simulink library "fixptlib"  (Simulink 4.00)
libraries: fixpt_lib_3p1 x25
settings Model: RequirementInfo=9  Creator=andyb  LastModifiedBy=andyb  ExtModeAutoUpdateStatusClock=off

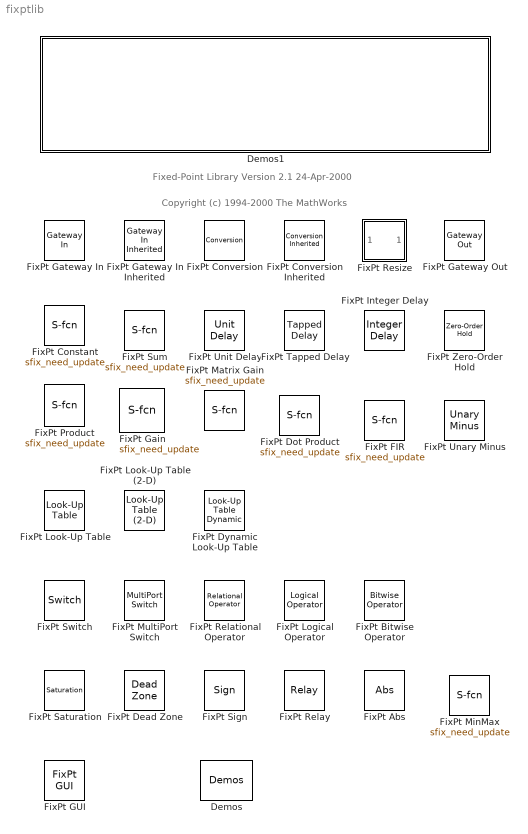
== system fixptlib ==
  note: Fixed-Point Library Version 2.1
      | 24-Apr-2000
  note: Copyright (c) 1994-2000 The MathWorks
  Demos : fixpt_lib_3p1/Demos
  Demos1 : Subsystem
      settings: OpenFcn=fixpt;  RTWFcnNameOpts=Auto  RTWFileNameOpts=Auto
      mask Display: disp('Obsolete version of Fixed-Point Blockset library.\n\nDouble Click this block to execute FIXPT.\n\nFIXPT will open latest version of the library.')
  FixPt Abs : fixpt_lib_3p1/Math/Abs  DoSatur=off
  FixPt Bitwise Operator : fixpt_lib_3p1/Bits/Bitwise Operator  logicop=AND  UseBitMask=on  BitMask=2^5+2^2+2^0  BitMaskRealWorld=Stored Integer
  FixPt Constant : S-Function  FunctionName=sfix_need_update  Parameters=NumInputs  PortCounts=[]  SFunctionModules=''  mask(Fixed-Point Constant (Obsolete)){constval=0.0, OutDataType=sfix(16), OutScaling=2^-1000, ConRadixGroup=Best Precision: Vector-wise, DblOver=off, SpecifyOutputDataType=on, SpecifyOutputScaling=on}
      mask prompts: constval "Constant value:"; OutDataType "Output data type:     ex.  sfix(16),  uint(8),  float('single')"; OutScaling "Output scaling:    Slope or [Slope Bias]    ex.  2^-9"; ConRadixGroup "Output scaling:"; DblOver "Override data type(s) with doubles"; SpecifyOutputDataType "Specify Output Data Type (otherwise inherit) ..."; SpecifyOutputScaling "Specify Output Scaling (otherwise inherit) ..."
      mask help:
      | Generate a constant value.
      |
      | This block is obsolete and is not compatible with the current version of Fixed Point Blockset.  The block needs to be replaced using FIXPT_UPDATE.
      mask init:
      | NumInputs = ~SpecifyOutputDataType | ~SpecifyOutputScaling;
      mask Help: This block is obsolete and is not compatible with the current version of Fixed Point Blockset.  The block needs to be replaced using FIXPT_UPDATE.
      mask StyleString: edit,edit,edit,popup(Use Specified Scaling|Best Precision: Vector-wise),checkbox,checkbox,checkbox
      mask CallbackString: fixptdialog(gcbh)|fixptdialog(gcbh)||fixptdialog(gcbh)|||
      mask Display:
      | disp(fixpt_mask_disp_prep(constval))
      | patch([2 2 10 10 4 4 8 8 4 4 2 ],[2 10 10 8 8 6 6 4 4 2 2 ],[0 0 0],'bottom-right');
  FixPt Conversion : fixpt_lib_3p1/Data Type/Conversion  ConvertRealWorld=Real World Value  OutputDataTypeScalingMode=Specify via dialog  OutDataType=sfix(16)  OutScaling=2^-10  DoSatur=off  DblOver=off  dolog=on
  FixPt Conversion Inherited : fixpt_lib_3p1/Data Type/Conversion Inherited  ConvertRealWorld=Real World Value  DoSatur=off  DblOver=off  dolog=on
  FixPt Dead Zone : fixpt_lib_3p1/Nonlinear/Dead Zone  UpperValue=1  LowerValue=-1  DoSatur=off
  FixPt Dot Product : S-Function  FunctionName=sfix_need_update  Parameters=2  PortCounts=[]  SFunctionModules=''  mask(Fixed-Point Dot Product (Obsolete)){OutDataType=sfix(16), OutScaling=2^-10, LockScale=off, RndMeth=Floor, DoSatur=off, DblOver=off, dolog=on, SpecifyOutputDataTypeAndScaling=on}
      mask prompts: OutDataType "Output data type:     ex.  sfix(16),  uint(8),  float('single')"; OutScaling "Output scaling:    Slope or [Slope Bias]    ex.  2^-9"; LockScale "Lock output scaling so autoscaling tool can't change it"; RndMeth "Round toward:"; DoSatur "Saturate to max or min when overflows occur"; DblOver "Override data type(s) with doubles"; dolog "Log minimums and maximums"
      mask help:
      | Inner (dot) product.
      | y = sum(conj(u1).*u2)
      |
      | This block is obsolete and is not compatible with the current version of Fixed Point Blockset.  The block needs to be replaced using FIXPT_UPDATE.
      mask Help: This block is obsolete and is not compatible with the current version of Fixed Point Blockset.  The block needs to be replaced using FIXPT_UPDATE.
      mask StyleString: edit,edit,checkbox,popup(Zero|Nearest|Ceiling|Floor),checkbox,checkbox,checkbox,checkbox
      mask CallbackString: fixptdialog(gcbh)|||||||
      mask Display:
      | patch([0.55 0.5433 0.525 0.5 0.475 0.4567 0.45 0.4567 0.475 0.5 0.525 0.5433 0.55],[ 0.5 0.525 0.5433 0.55 0.5433 0.525 0.5 0.475 0.4567 0.45 0.4567 0.475 0.5],[0 0 0])
      | patch([2 2 10 10 4 4 8 8 4 4 2 ],[2 10 10 8 8 6 6 4 4 2 2 ],[0 0 0],'bottom-right');
  FixPt Dynamic Look-Up Table : fixpt_lib_3p1/LookUp/Look-Up Table Dynamic  LookUpMeth=Interpolation-Use End Values  OutputDataTypeScalingMode=Specify via dialog  OutDataType=sfix(16)  OutScaling=2^-10  DoSatur=off  DblOver=off  dolog=on
  FixPt FIR : S-Function  FunctionName=sfix_need_update  Parameters=1  PortCounts=[]  SFunctionModules=''  mask(Fixed-Point FIR (Obsolete)){mgainval=[0.1:0.1:1 0.9:-0.1:0.1], vinit=0.0, samptime=-1, GainDataType=sfix( 16 ), GainScaling=2^-14, MatRadixGroup=Best Precision: Matrix-wise, OutDataType=sfix(16), OutScaling=2^-10, LockScale=off, RndMeth=Floor, DoSatur=off, DblOver=off, dolog=on, SpecifyOutputDataTypeAndScaling=on}
      mask prompts: mgainval "FIR coefficients:"; vinit "Initial condition:"; samptime "Sample time:"; GainDataType "Parameter data type:     ex. sfix(16),  uint(8), float('single')"; GainScaling "Parameter scaling:    Slope    ex.  2^-9"; MatRadixGroup "Parameter scaling:"; OutDataType "Output data type:     ex.  sfix(16),  uint(8),  float('single')"; OutScaling "Output scaling:    Slope or [Slope Bias]    ex.  2^-9"; LockScale "Lock output scaling so autoscaling tool can't change it"; RndMeth "Round toward:"; DoSatur "Saturate to max or min when overflows occur"; DblOver "Override data type(s) with doubles"; dolog "Log minimums and maximums"
      mask help:
      | Implement a finite impulse response (FIR) filter.
      |
      | This block is obsolete and is not compatible with the current version of Fixed Point Blockset.  The block needs to be replaced using FIXPT_UPDATE.
      mask init:
      | if MatRadixGroup == 5
      |     RadixGroup = 1; % BEST_PREC_MAT
      | elseif MatRadixGroup == 4
      |     RadixGroup = 2; % BEST_PREC_COL
      | elseif MatRadixGroup == 3
      |     RadixGroup = 3; % BEST_PREC_ROW
      | elseif MatRadixGroup == 2
      |     RadixGroup = 4; % BEST_PREC_ELE
      | else
      |     RadixGroup = 0; % BEST_PREC_OFF
      | end
      mask Help: This block is obsolete and is not compatible with the current version of Fixed Point Blockset.  The block needs to be replaced using FIXPT_UPDATE.
      mask StyleString: edit,edit,edit,edit,edit,popup(Use Specified Scaling|Best Precision: Element-wise|Best Precision: Row-wise|Best Precision: Column-wise|Best Precision: Matrix-wise),edit,edit,checkbox,popup(Zero|Nearest|Ceiling|Floor),checkbox,checkbox,checkbox,checkbox
      mask CallbackString: fixptdialog(gcbh)|||fixptdialog(gcbh)||fixptdialog(gcbh)|fixptdialog(gcbh)|||||||
      mask Display:
      | fprintf(fixpt_fir_mask_data(mgainval,'dispstr'))
      | plot(fixpt_fir_mask_data(mgainval,1),fixpt_fir_mask_data(mgainval,0))
      | patch([2 2 10 10 4 4 8 8 4 4 2 ],[2 10 10 8 8 6 6 4 4 2 2 ],[0 0 0],'bottom-right');
  FixPt GUI : fixpt_lib_3p1/FixPt GUI
  FixPt Gain : S-Function  FunctionName=sfix_need_update  Parameters=1  PortCounts=[]  SFunctionModules=''  mask(Fixed-Point Gain (Obsolete)){gainval=1.0, GainDataType=sfix( 16 ), GainScaling=2^-14, VecRadixGroup=Best Precision: Matrix-wise, OutDataType=sfix(16), OutScaling=2^-10, LockScale=off, RndMeth=Floor, DoSatur=off, DblOver=off, dolog=on, ElevsMatrix=Element-wise(K.*u), SpecifyOutputDataTypeAndScaling=on}
      mask prompts: gainval "Gain value:"; GainDataType "Parameter data type:     ex. sfix(16),  uint(8), float('single')"; GainScaling "Parameter scaling:    Slope    ex.  2^-9"; VecRadixGroup "Parameter scaling:"; OutDataType "Output data type:     ex.  sfix(16),  uint(8),  float('single')"; OutScaling "Output scaling:    Slope or [Slope Bias]    ex.  2^-9"; LockScale "Lock output scaling so autoscaling tool can't change it"; RndMeth "Round toward:"; DoSatur "Saturate to max or min when overflows occur"; DblOver "Override data type(s) with doubles"; dolog "Log minimums and maximums"; ElevsMatrix "Multiplication"
      mask help:
      | Multiply the input by a constant (gain).
      |
      | This block is obsolete and is not compatible with the current version of Fixed Point Blockset.  The block needs to be replaced using FIXPT_UPDATE.
      mask init:
      | if VecRadixGroup >= 5
      |     RadixGroup = 1; % BEST_PREC_MAT
      | elseif VecRadixGroup == 4
      |     RadixGroup = 2; % BEST_PREC_COL
      | elseif VecRadixGroup == 3
      |     RadixGroup = 3; % BEST_PREC_ROW
      | elseif VecRadixGroup == 2
      |     RadixGroup = 4; % BEST_PREC_ELE
      | else
      |     RadixGroup = 0; % BEST_PREC_OFF
      | end
      mask Help: This block is obsolete and is not compatible with the current version of Fixed Point Blockset.  The block needs to be replaced using FIXPT_UPDATE.
      mask StyleString: edit,edit,edit,popup(Use Specified Scaling|Best Precision: Element-wise|Best Precision: Row-wise|Best Precision: Column-wise|Best Precision: Matrix-wise|Best Precision: Vector-wise),edit,edit,checkbox,popup(Zero|Nearest|Ceiling|Floor),checkbox,checkbox,checkbox,popup(Element-wise(K.*u)|Matrix(K*u)|Matrix(u*K)|Matrix(K*u) (u vector)),checkbox
      mask CallbackString: fixptdialog(gcbh)|fixptdialog(gcbh)||fixptdialog(gcbh)|fixptdialog(gcbh)||||||||
      mask Display:
      | disp(fixpt_mask_disp_prep(gainval))
      | plot(fixpt_gain_mask_data(gcbh,1),fixpt_gain_mask_data(gcbh,0))
      | patch([2 2 10 10 4 4 8 8 4 4 2 ],[2 10 10 8 8 6 6 4 4 2 2 ],[0 0 0],'bottom-right');
  FixPt Gateway In : fixpt_lib_3p1/Data Type/Gateway In  InRealWorld=Real World Value  OutputDataTypeScalingMode=Specify via dialog  OutDataType=sfix(16)  OutScaling=2^-10  DoSatur=off  DblOver=off  dolog=on
  FixPt Gateway In Inherited : fixpt_lib_3p1/Data Type/Gateway In Inherited  InRealWorld=Real World Value  DoSatur=off  DblOver=off  dolog=on
  FixPt Gateway Out : fixpt_lib_3p1/Data Type/Gateway Out  OutRealWorld=Real World Value  OutBuiltInType=double  DoSatur=off  dolog=off
  FixPt Integer Delay : fixpt_lib_3p1/Delays & Holds/Integer Delay  vinit=0.0  samptime=-1  NumDelays=4
  FixPt Logical Operator : fixpt_lib_3p1/Logic & Comparison/Logical Operator  logicop=AND  NumInputPorts=2  LogicDataType=uint(8)
  FixPt Look-Up Table : fixpt_lib_3p1/LookUp/Look-Up Table  XLookUpData=-5:5  YLookUpData=tanh([-5:5])  LookUpMeth=Interpolation-Use End Values  OutputDataTypeScalingMode=Specify via dialog  OutDataType=sfix(16)  OutScaling=2^-10  DoSatur=off  DblOver=off  dolog=on
  FixPt Look-Up Table (2-D) : fixpt_lib_3p1/LookUp/Look-Up Table (2-D)  RowLookUpData=[1:3]  ColLookUpData=[1:3]  TableLookUpData=[4 5 6;16 19 20;10 18 23]  LookUpMeth=Interpolation-Use End Values  OutputDataTypeScalingMode=Specify via dialog  OutDataType=sfix(16)  OutScaling=2^-10  DoSatur=off  DblOver=off  dolog=on
  FixPt Matrix Gain : S-Function  FunctionName=sfix_need_update  Parameters=1  PortCounts=[]  SFunctionModules=''  mask(Fixed-Point Matrix Gain (Obsolete)){mgainval=eye(3,3), GainDataType=sfix( 16 ), GainScaling=2^-14, MatRadixGroup=Best Precision: Matrix-wise, OutDataType=sfix(16), OutScaling=2^-10, LockScale=off, RndMeth=Floor, DoSatur=off, DblOver=off, dolog=on, ElevsMatrix=Matrix(K*u) (u vector), SpecifyOutputDataTypeAndScaling=on}
      mask prompts: mgainval "Gain matrix value:"; GainDataType "Parameter data type:     ex. sfix(16),  uint(8), float('single')"; GainScaling "Parameter scaling:    Slope    ex.  2^-9"; MatRadixGroup "Parameter scaling:"; OutDataType "Output data type:     ex.  sfix(16),  uint(8),  float('single')"; OutScaling "Output scaling:    Slope or [Slope Bias]    ex.  2^-9"; LockScale "Lock output scaling so autoscaling tool can't change it"; RndMeth "Round toward:"; DoSatur "Saturate to max or min when overflows occur"; DblOver "Override data type(s) with doubles"; dolog "Log minimums and maximums"; ElevsMatrix "Multiplication"
      mask help:
      | Multiply the input by a constant (gain).
      |
      | This block is obsolete and is not compatible with the current version of Fixed Point Blockset.  The block needs to be replaced using FIXPT_UPDATE.
      mask init: same as fixptlib/FixPt FIR
      mask Help: This block is obsolete and is not compatible with the current version of Fixed Point Blockset.  The block needs to be replaced using FIXPT_UPDATE.
      mask StyleString: edit,edit,edit,popup(Use Specified Scaling|Best Precision: Element-wise|Best Precision: Row-wise|Best Precision: Column-wise|Best Precision: Matrix-wise),edit,edit,checkbox,popup(Zero|Nearest|Ceiling|Floor),checkbox,checkbox,checkbox,popup(Element-wise(K.*u)|Matrix(K*u)|Matrix(u*K)|Matrix(K*u) (u vector)),checkbox
      mask CallbackString: fixptdialog(gcbh)|fixptdialog(gcbh)||fixptdialog(gcbh)|fixptdialog(gcbh)||||||||
      mask Display:
      | fprintf('K')
      | patch([2 2 10 10 4 4 8 8 4 4 2 ],[2 10 10 8 8 6 6 4 4 2 2 ],[0 0 0],'bottom-right');
  FixPt MinMax : S-Function  FunctionName=sfix_need_update  Parameters=Inputs  PortCounts=[]  SFunctionModules=''  mask(Fixed-Point MinMax (Obsolete)){Function=min, Inputs=1, OutDataType=sfix(16), OutScaling=2^-10, LockScale=off, RndMeth=Floor, DoSatur=off, DblOver=off, dolog=on, SpecifyOutputDataTypeAndScaling=on}
      mask prompts: Inputs "Number of input ports:"; OutDataType "Output data type:     ex.  sfix(16),  uint(8),  float('single')"; OutScaling "Output scaling:    Slope or [Slope Bias]    ex.  2^-9"; LockScale "Lock output scaling so autoscaling tool can't change it"; RndMeth "Round toward:"; DoSatur "Saturate to max or min when overflows occur"; DblOver "Override data type(s) with doubles"; dolog "Log minimums and maximums"
      mask help:
      | Output min or max of input.  For a single input, operators are applied across the input vector.  For multiple inputs, operators are applied across the inputs.
      |
      | This block is obsolete and is not compatible with the current version of Fixed Point Blockset.  The block needs to be replaced using FIXPT_UPDATE.
      mask Help: This block is obsolete and is not compatible with the current version of Fixed Point Blockset.  The block needs to be replaced using FIXPT_UPDATE.
      mask StyleString: popup(min|max),edit,edit,edit,checkbox,popup(Zero|Nearest|Ceiling|Floor),checkbox,checkbox,checkbox,checkbox
      mask CallbackString: ||fixptdialog(gcbh)|||||||
      mask Display:
      | disp(char((Function==1)*'min'+(Function==2)*'max'))
      | patch([2 2 10 10 4 4 8 8 4 4 2 ],[2 10 10 8 8 6 6 4 4 2 2 ],[0 0 0],'bottom-right');
  FixPt MultiPort Switch : fixpt_lib_3p1/Select/MultiPort Switch  NumInputPorts=3  zeroidx=off  DoSatur=off  dolog=on
  FixPt Product : S-Function  FunctionName=sfix_need_update  Parameters=length(mulstr)  PortCounts=[]  SFunctionModules=''  mask(Fixed-Point Product (Obsolete)){listofops=**, OutDataType=sfix(16), OutScaling=2^-10, LockScale=off, RndMeth=Floor, DoSatur=off, DblOver=off, dolog=on, ElevsMatrix=Element-wise(.*), SpecifyOutputDataTypeAndScaling=on}
      mask prompts: listofops "Enter */ characters or the number of inputs:"; OutDataType "Output data type:     ex.  sfix(16),  uint(8),  float('single')"; OutScaling "Output scaling:    Slope or [Slope Bias]    ex.  2^-9"; LockScale "Lock output scaling so autoscaling tool can't change it"; RndMeth "Round toward:"; DoSatur "Saturate to max or min when overflows occur"; DblOver "Override data type(s) with doubles"; dolog "Log minimums and maximums"; ElevsMatrix "Multiplication"
      mask help:
      | Multiply or divide inputs. Specify one of the following:
      | a)  A * or / for each input
      | b)  The number of inputs if only multiplication is desired
      | c)  A single * or / to collapse a vector
      |
      | This block is obsolete and is not compatible with the current version of Fixed Point Blockset.  The block needs to be replaced using FIXPT_UPDATE.
      mask init:
      | mulstr = '**';
      | if ~isempty (listofops)
      |    if all(  ( listofops == '*' ) | ( listofops == '/' )  )
      |       mulstr = listofops;
      |    else
      |       i = eval(listofops,'-1');
      |       if i < 2
      |          mulstr = '*';
      |          if i < 1
      |            disp(get_param(gcb,'Name'))
      |            disp('Error: Please enter multiplier/divider string OR number of inputs');
      |          end
      |       else
      |          i = min(i,15);
      |          mulstr(1:i ) = '*';
      |       end
      |    end
      | end
      | if ElevsMatrix == 2
      |   MatrixMult=1;
      | else
      |   MatrixMult=0;
      | end
      mask Help: This block is obsolete and is not compatible with the current version of Fixed Point Blockset.  The block needs to be replaced using FIXPT_UPDATE.
      mask StyleString: edit,edit,edit,checkbox,popup(Zero|Nearest|Ceiling|Floor),checkbox,checkbox,checkbox,popup(Element-wise(.*)|Matrix(*)),checkbox
      mask CallbackString: |fixptdialog(gcbh)||||||||
      mask Display:
      | plot(fixpt_mul_mask_data(gcbh,mulstr,1,MatrixMult),fixpt_mul_mask_data(gcbh,mulstr,0,MatrixMult))
      | patch([2 2 10 10 4 4 8 8 4 4 2 ],[2 10 10 8 8 6 6 4 4 2 2 ],[0 0 0],'bottom-right');
      | disp(fixpt_mul_mask_data_str(gcbh,MatrixMult))
  FixPt Relational Operator : fixpt_lib_3p1/Logic & Comparison/Relational Operator  relop=<=  LogicDataType=uint(8)
  FixPt Relay : fixpt_lib_3p1/Nonlinear/Relay  OnSwitchValue=0  OffSwitchValue=0  OnOutputValue=1  OffOutputValue=0  OutputDataTypeScalingMode=Specify via dialog  OutDataType=uint(8)  OutScaling=2^-10  ConRadixGroup=Best Precision: Vector-wise  DblOver=off
  FixPt Resize : Subsystem  mask(Fixed-Point to Fixed-Point Resize (Obsolete)){ResizeAction=Decrease bits by half, RetainRangeOrPrecision=range, NumBits=16, RndMeth=Floor, DoSatur=off, DblOver=off, dolog=off}
      mask prompts: ResizeAction "Resize action:"; RetainRangeOrPrecision "Retain:"; NumBits "Number of Bits"; RndMeth "Round toward:"; DoSatur "Saturate to max or min when overflows occur"; DblOver "Override data type(s) with doubles"; dolog "Log minimums and maximums"
      mask help:
      | Resize the number of bits used by a Fixed-Point Blockset signal.
      |
      | This block is obsolete and is not compatible with the current version of Fixed Point Blockset.  The block needs to be replaced using FIXPT_UPDATE.
      settings: RTWFcnNameOpts=Auto  RTWFileNameOpts=Auto
      mask Help: This block is obsolete and is not compatible with the current version of Fixed Point Blockset.  The block needs to be replaced using FIXPT_UPDATE.
      mask StyleString: popup(Decrease bits by half|Decrease bits by specified number|Increase bits by twice|Increase bits by specified number|Set bits to specified number),popup(range|precision),edit,popup(Zero|Nearest|Ceiling|Floor),checkbox,checkbox,checkbox
      mask CallbackString: if any(strcmp(get_param(gcb, 'ResizeAction'), {'Decrease bits by half', 'Increase bits by twice'})), set_param(gcb, 'MaskVisibilities', {'on'; 'on'; 'off'; 'on'; 'on'; 'on'; 'on'}), else, set_param(gcb, 'MaskVisibilities', {'on'; 'on'; 'on'; 'on'; 'on'; 'on'; 'on'}), end||||||
      mask Display:
      | fprintf('Resize')
      | patch([0.725 0.725 0.975 0.975 0.8 0.8 0.925 0.925 0.8 0.8 0.725 ],[0.025 0.275 0.275 0.2 0.2 0.15 0.15 0.075 0.075 0.025 0.025 ],[0 0 0]);
      | patch([0.05 0.05 0.3 0.3 0.125 0.125 0.25 0.25 0.125 0.125 0.05 ],[0.7 0.95 0.95 0.875 0.875 0.825 0.825 0.75 0.75 0.7 0.7 ],[0 0 0]);
  FixPt Saturation : fixpt_lib_3p1/Nonlinear/Saturation  uplimit=0.5  lowlimit=-0.5
  FixPt Sign : fixpt_lib_3p1/Nonlinear/Sign
  FixPt Sum : S-Function  FunctionName=sfix_need_update  Parameters=Inputs  PortCounts=[]  SFunctionModules=''  mask(Fixed-Point Sum (Obsolete)){listofsigns=++, OutDataType=sfix(16), OutScaling=2^-10, LockScale=off, RndMeth=Floor, DoSatur=off, DblOver=off, dolog=on, SpecifyOutputDataTypeAndScaling=on}
      mask prompts: listofsigns "Enter +- characters or the number of inputs:"; OutDataType "Output data type:     ex.  sfix(16),  uint(8),  float('single')"; OutScaling "Output scaling:    Slope or [Slope Bias]    ex.  2^-9"; LockScale "Lock output scaling so autoscaling tool can't change it"; RndMeth "Round toward:"; DoSatur "Saturate to max or min when overflows occur"; DblOver "Override data type(s) with doubles"; dolog "Log minimums and maximums"
      mask help:
      | Add or subtract inputs. Specify one of the following:
      | a)  A + or - for each input
      | b)  The number of inputs if only addition is desired
      | c)  A single + or - to collapse a vector
      |
      | This block is obsolete and is not compatible with the current version of Fixed Point Blockset.  The block needs to be replaced using FIXPT_UPDATE.
      mask init:
      | addstr = '++';
      | if ~isempty (listofsigns)
      |    if all(  ( listofsigns == '+' ) | ( listofsigns == '-' )  )
      |       addstr = listofsigns;
      |    else
      |       Inputs=eval(listofsigns,'-1');
      |       if Inputs < 2
      |          addstr = '+';
      |          if Inputs < 1
      |            disp(get_param(gcb,'Name'))
      |            disp('Error: must enter plus/minus string OR number of inputs');
      |          end
      |       else
      |          Inputs = min(Inputs,15);
      |          addstr(1:Inputs ) = '+';
      |       end
      |    end
      | end
      | Inputs = length(addstr);
      mask Help: This block is obsolete and is not compatible with the current version of Fixed Point Blockset.  The block needs to be replaced using FIXPT_UPDATE.
      mask StyleString: edit,edit,edit,checkbox,popup(Zero|Nearest|Ceiling|Floor),checkbox,checkbox,checkbox,checkbox
      mask CallbackString: |fixptdialog(gcbh)|||||||
      mask Display:
      | plot(fixpt_mul_mask_data(gcbh,addstr,1,0),fixpt_mul_mask_data(gcbh,addstr,0,0))
      | patch([2 2 10 10 4 4 8 8 4 4 2 ],[2 10 10 8 8 6 6 4 4 2 2 ],[0 0 0],'bottom-right');
  FixPt Switch : fixpt_lib_3p1/Select/Switch  Criteria=u2 >= Threshold  vthresh=0.5  DoSatur=off  dolog=on
  FixPt Tapped Delay : fixpt_lib_3p1/Delays & Holds/Tapped Delay  vinit=0.0  samptime=-1  NumDelays=4  DelayOrder=Oldest
  FixPt Unary Minus : fixpt_lib_3p1/Math/Unary Minus  DoSatur=off
  FixPt Unit Delay : fixpt_lib_3p1/Delays & Holds/Unit Delay  vinit=0.0  samptime=-1
  FixPt Zero-Order Hold : fixpt_lib_3p1/Delays & Holds/Zero-Order Hold  samptime=1.0

== system fixptlib/Demos1 ==

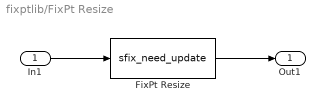
== system fixptlib/FixPt Resize ==
  In1 : Inport  Port=1  LatchInput=off
  FixPt Resize : S-Function  FunctionName=sfix_need_update  Parameters=1  PortCounts=[]  SFunctionModules=''
  Out1 : Outport  Port=1
  wires:
  In1/1 -> FixPt Resize/1
  FixPt Resize/1 -> Out1/1
